simulink model "helicopter_breach"  (R2018b)
settings: Solver=FixedStepAuto  StartTime=0.0  StopTime=4.0  FixedStep=0.01  RelTol=1e-3
undefined symbols (not defined in the file): a, i, K, options
libraries: simulink x2
settings Model: Creator=alex  LastModifiedBy=kekatos
settings DataIOCC: LimitDataPoints=on  SaveFormat=Array
settings OptimizationCC: LifeSpan=inf
settings DebuggingCC: SFUnexpectedBacktrackingDiag=warning  SFNoUnconditionalDefaultTransitionDiag=warning  SFExecutionAtInitializationDiag=none
settings HardwareCC: ProdBitPerPointer=32  ProdBitPerSizeT=32  ProdBitPerPtrDiffT=32  ProdLargestAtomicFloat=None  ProdIntDivRoundTo=Undefined  ProdEndianess=Unspecified  ProdWordSize=32  ProdHWDeviceType=32-bit Generic
settings ModelReferenceCC: PropagateSignalLabelsOutOfModel=off
settings SFSimCC: SimUseLocalCustomCode=off
settings RTWCC: RTWUseLocalCustomCode=off
settings CodeAppCC: StateflowObjectComments=on
settings GRTTargetCC: TargetLangStandard=C89/C90 (ANSI)  GeneratePreprocessorConditionals=Disable all
settings ConfigComp: CovMetricSettings=dw  CovHtmlReporting=on  CovSaveCumulativeToWorkspaceVar=on  CovSaveSingleToWorkspaceVar=on  CovExternalEMLEnable=off  CovSFcnEnable=off

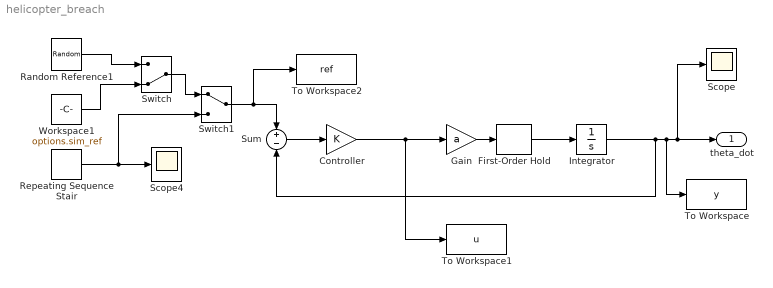
== system helicopter_breach ==
  "Controller " : Gain  Gain=K
  First-Order Hold : simulink/Discrete/First-Order Hold  DisableCoverage=on  Ts=options.dt
      settings: SourceProductName=Simulink  SourceProductBaseCode=SL
  Gain : Gain  Gain=a
  Integrator : Integrator  InitialCondition=i
  Random Reference1 : UniformRandomNumber  Minimum=options.ref_min  Maximum=options.ref_max  Seed=randi(2^32,[1 ])  SampleTime=options.ref_Ts
  Repeating Sequence Stair : simulink/Sources/Repeating Sequence Stair  OutValues=options.sim_cov  tsamp=options.ref_Ts  OutMin=[]  OutMax=[]  OutDataTypeStr=double  OutputDataTypeScalingMode=double  OutDataType=fixdt(0,8)  ConRadixGroup=Best Precision: Vector-wise  OutScaling=2^-12
  Scope : Scope
  Scope4 : Scope
  Sum : Sum  Inputs=+-
  Switch : ManualSwitch  CurrentSetting=0
  Switch1 : ManualSwitch
  To Workspace : ToWorkspace  VariableName=y  SaveFormat=Structure With Time  SampleTime=-1
  To Workspace1 : ToWorkspace  VariableName=u  SaveFormat=Structure With Time  SampleTime=-1
  To Workspace2 : ToWorkspace  VariableName=ref  SaveFormat=Structure With Time  SampleTime=options.dt
  Workspace1 : Constant  InitFcn=|  Value=options.sim_ref
      | K = 10;
      | i = 0; 
      | a = 1;
  theta_dot : Outport
  wires:
  Gain/1 -> First-Order Hold/1
  Integrator/1 -> Sum/2, To Workspace/1, Scope/1, theta_dot/1
  "Controller "/1 -> To Workspace1/1, Gain/1
  Switch1/1 -> To Workspace2/1, Sum/1
  Sum/1 -> "Controller "/1
  Workspace1/1 -> Switch/2
  Repeating Sequence Stair/1 -> Scope4/1, Switch1/2
  Random Reference1/1 -> Switch/1
  Switch/1 -> Switch1/1
  First-Order Hold/1 -> Integrator/1
